simulink model "invBridge120"  (R2026a)
settings: Solver=FixedStepDiscrete  StopTime=0.1  FixedStep=ip.Ts_power
model workspace (MATLAB code in the model file):
  | ip = invParams();
libraries: nesl_utility x18, fl_lib x13, ee_lib x3
settings Model: Creator=phamn  LastModifiedBy=phamn
settings SimscapeCC: SimscapeLogType=none

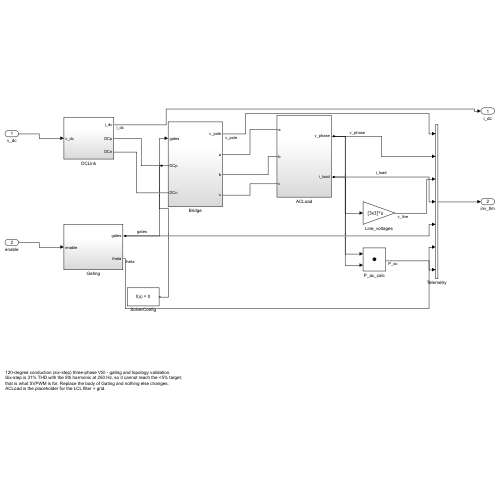
[thumbnail: Simulink's stored preview of the top-level diagram]
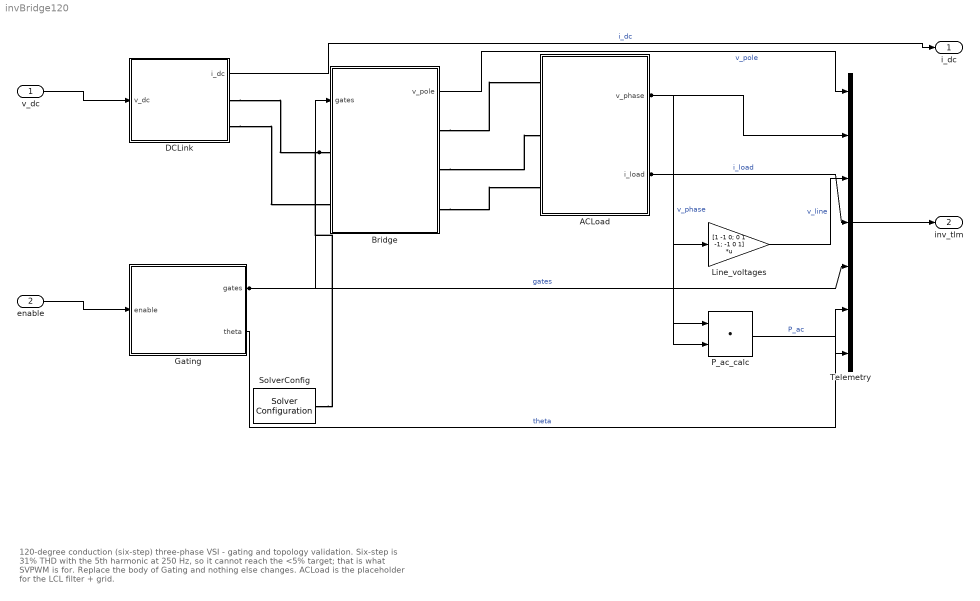
== system invBridge120 ==
  note: 120-degree conduction (six-step) three-phase VSI - gating and topology validation.
      | Six-step is 31% THD with the 5th harmonic at 250 Hz, so it cannot reach the <5% target;
      | that is what SVPWM is for. Replace the body of Gating and nothing else changes.
      | ACLoad is the placeholder for the LCL filter + grid.
  v_dc : Inport
  enable : Inport  Port=2
  ACLoad : Subsystem
  Bridge : Subsystem
  DCLink : Subsystem
  Gating : Subsystem
  Line_voltages : Gain  Gain=[1 -1 0; 0 1 -1; -1 0 1]  Multiplication=Matrix(K*u)
  P_ac_calc : DotProduct  OutDataTypeStr=Inherit: Inherit via internal rule
  SolverConfig : nesl_utility/Solver Configuration  PhysicalDomain=network_engine_domain  SubClassName=solver  LeftPortType=input  RightPortType=generic  Tones=[]  Harmonics=[]  SimulateNoise=off  Profile=off  UseLocalSampling=off  EnableSwitchedLinearOptims=on  FrequencyDomain=off  UseCCode=off  RelTol=0.001  AbsTol=0.001  MinStep=1e-09  ToWorkspace=off  RevertToSquareIcSolve=off  NumHomotopyIterations=100  PhasorMode=off  PhasorModeNumHarmonics=1  ConsistencySolver=NEWTON_XTOL_AFTER_FTOL  CanonicalOrdering=CANONICAL  OptimizeIntermediates=OPTIMIZED  IndexReductionMethod=DerivativeReplacement  DoDC=off  ResidualTolerance=1e-09  ConsistencyTolSource=GLOBAL  ConsistencyAbsTol=0.001  ConsistencyRelTol=0.001  ConsistencyTolFactor=0.001  UseLocalSolver=on  LocalSolverChoice=NE_BACKWARD_EULER_ADVANCER  ResolveIndetEquations=on  FunctionEvalNumThread=1  LocalSolverSampleTime=ip.Ts_power  DoFixedCost=off  MaxNonlinIter=3  MaxModeIter=2  ComputeImpulses=off  ImpulseIterations=2  LinearAlgebra=auto  LinearAlgebraNumThread=0  EquationFormulation=NE_TIME_EF  DelaysMemoryBudget=1024  AutomaticFiltering=on  FilteringTimeConstant=0.001  PartitionStorageMethod=AS_NEEDED  PartitionMemoryBudget=1024  PartitionMethod=ROBUST  MultibodyUseLocalSolver=off  MultibodyLocalSolverChoice=ODE1  MultibodyLocalSolverSampleTime=0.001
  Telemetry : BusCreator  Inputs=7
  i_dc : Outport
  inv_tlm : Outport  Port=2
  wires:
  v_dc/1 -> DCLink/1(v_dc)
  enable/1 -> Gating/1(enable)
  Gating/1(gates) -> Bridge/1(gates), Telemetry/5  "gates"
  Gating/2(theta) -> Telemetry/6  "theta"
  Bridge/1(v_pole) -> Telemetry/1  "v_pole"
  ACLoad/1(v_phase) -> Telemetry/2, Line_voltages/1, P_ac_calc/1  "v_phase"
  ACLoad/2(i_load) -> Telemetry/4, P_ac_calc/2  "i_load"
  Line_voltages/1 -> Telemetry/3  "v_line"
  P_ac_calc/1 -> Telemetry/7  "P_ac"
  DCLink/1(i_dc) -> i_dc/1  "i_dc"
  Telemetry/1 -> inv_tlm/1
  connections:
  Bridge/LConn1 -- DCLink/RConn1 -- SolverConfig/RConn1
  DCLink/RConn2 -- Bridge/LConn2
  Bridge/RConn1 -- ACLoad/LConn1
  Bridge/RConn2 -- ACLoad/LConn2
  Bridge/RConn3 -- ACLoad/LConn3

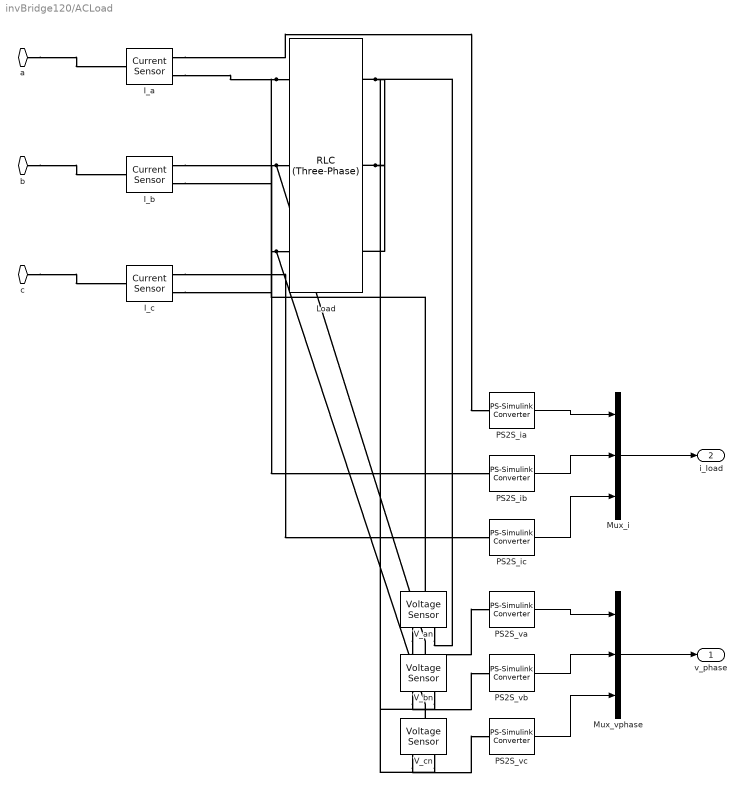
== system invBridge120/ACLoad ==
  I_a : fl_lib/Electrical/Electrical Sensors/Current Sensor
  I_b : fl_lib/Electrical/Electrical Sensors/Current Sensor
  I_c : fl_lib/Electrical/Electrical Sensors/Current Sensor
  Load : ee_lib/Passive/RLC Assemblies/RLC (Three-Phase)  port_option=ee.enum.threePhasePort.expanded  component_structure=ee.enum.rlc.structure.R  R=ip.R_load Ohm  L=ip.L_load H  C=ip.Cf F  R_parasitic=0 Ohm  G_parasitic=0 1/Ohm  IL_specify=off  IL_priority=High  IL=[0, 0, 0] A  IL_nominal_specify=off  IL_nominal_value=1  IL_nominal_unit=A  VC_specify=off  VC_priority=High  VC=[0, 0, 0] V  VC_nominal_specify=off  VC_nominal_value=1  VC_nominal_unit=V
  Mux_i : Mux  Inputs=3
  Mux_vphase : Mux  Inputs=3
  PS2S_ia : nesl_utility/PS-Simulink Converter  PhysicalDomain=network_engine_domain  SubClassName=ps_output  LeftPortType=input  RightPortType=output  PseudoPeriodic=off  Frequencies=[]  VectorFormat=inherit  Unit=inherit  AffineConversion=off
  PS2S_ib : nesl_utility/PS-Simulink Converter  PhysicalDomain=network_engine_domain  SubClassName=ps_output  LeftPortType=input  RightPortType=output  PseudoPeriodic=off  Frequencies=[]  VectorFormat=inherit  Unit=inherit  AffineConversion=off
  PS2S_ic : nesl_utility/PS-Simulink Converter  PhysicalDomain=network_engine_domain  SubClassName=ps_output  LeftPortType=input  RightPortType=output  PseudoPeriodic=off  Frequencies=[]  VectorFormat=inherit  Unit=inherit  AffineConversion=off
  PS2S_va : nesl_utility/PS-Simulink Converter  PhysicalDomain=network_engine_domain  SubClassName=ps_output  LeftPortType=input  RightPortType=output  PseudoPeriodic=off  Frequencies=[]  VectorFormat=inherit  Unit=inherit  AffineConversion=off
  PS2S_vb : nesl_utility/PS-Simulink Converter  PhysicalDomain=network_engine_domain  SubClassName=ps_output  LeftPortType=input  RightPortType=output  PseudoPeriodic=off  Frequencies=[]  VectorFormat=inherit  Unit=inherit  AffineConversion=off
  PS2S_vc : nesl_utility/PS-Simulink Converter  PhysicalDomain=network_engine_domain  SubClassName=ps_output  LeftPortType=input  RightPortType=output  PseudoPeriodic=off  Frequencies=[]  VectorFormat=inherit  Unit=inherit  AffineConversion=off
  V_an : fl_lib/Electrical/Electrical Sensors/Voltage Sensor
  V_bn : fl_lib/Electrical/Electrical Sensors/Voltage Sensor
  V_cn : fl_lib/Electrical/Electrical Sensors/Voltage Sensor
  a : PMIOPort  Side=Left
  b : PMIOPort  Port=2  Side=Left
  c : PMIOPort  Port=3  Side=Left
  v_phase : Outport
  i_load : Outport  Port=2
  wires:
  PS2S_ia/1 -> Mux_i/1
  PS2S_va/1 -> Mux_vphase/1
  PS2S_ib/1 -> Mux_i/2
  PS2S_vb/1 -> Mux_vphase/2
  PS2S_ic/1 -> Mux_i/3
  PS2S_vc/1 -> Mux_vphase/3
  Mux_i/1 -> i_load/1
  Mux_vphase/1 -> v_phase/1
  connections:
  a/RConn1 -- I_a/LConn1
  Load/LConn1 -- I_a/RConn2 -- V_an/LConn1
  I_a/RConn1 -- PS2S_ia/LConn1
  V_an/RConn2 -- V_bn/RConn2 -- V_cn/RConn2 -- Load/RConn1 -- Load/RConn2 -- Load/RConn3
  V_an/RConn1 -- PS2S_va/LConn1
  b/RConn1 -- I_b/LConn1
  Load/LConn2 -- I_b/RConn2 -- V_bn/LConn1
  I_b/RConn1 -- PS2S_ib/LConn1
  V_bn/RConn1 -- PS2S_vb/LConn1
  c/RConn1 -- I_c/LConn1
  Load/LConn3 -- I_c/RConn2 -- V_cn/LConn1
  I_c/RConn1 -- PS2S_ic/LConn1
  V_cn/RConn1 -- PS2S_vc/LConn1

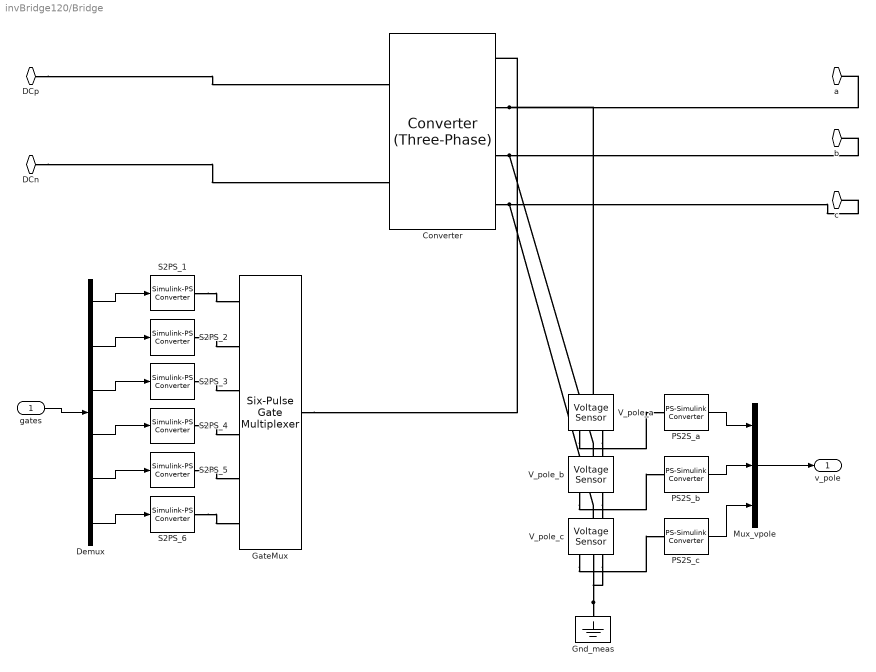
== system invBridge120/Bridge ==
  gates : Inport
  Converter : ee_lib/Semiconductors & Converters/Converters/Converter (Three-Phase)  port_option=ee.enum.threePhasePort.expanded  fidelity_option=ee.enum.converters.fidelity.detailed  device_type=ee.enum.converters.switchingdevice.igbt  showThermalPort=false  K=0  Vth=ip.Vth_gate V  Vgt=1 V  Vgt_off=-1 V  Ih=1 A  Vf=ip.Vf_dev V  Ron=ip.Ron_dev Ohm  Rds=0.001 Ohm  Goff=ip.Goff_dev 1/Ohm  Eon_scalar=22.86e-3 J  Eoff_scalar=17.14e-3 J  Eoff_natural_commutation=10e-3 J  Voff=300 V  Iout_scalar=600 A  onCurrentMeasDelay=0 s  useCurrentFromPreviousCycle=false  useVoltageFromPreviousCycle=false  diode_param=ee.enum.converters.protectiondiode.nodynamics  diode_Vf=ip.Vf_dev V  diode_Ron=ip.Ron_dev Ohm  diode_Goff=1e-5 1/Ohm  diode_C=50 nF  diode_iRM=-235 A  diode_iF=300 A  diode_idot=-50 A/us  diode_trr_param=ee.enum.converters.diodetrr.trr_factor  diode_trr_factor=3  diode_trr=15 us  diode_Qrr=1500 s*uA  diode_rec_loss_model=ee.enum.diode.reverseRecoveryModel.fixed  diode_ErecVal=0 J  diode_scaleWithIandV=false  diode_ErecMat=zeros(2, 3) J  diode_TjrecVec=[298.15, 398.15] K  diode_IfrecVec=[.1, 1, 10] A  diode_IrecVal=10 A  diode_VrecVal=10 V  diode_tFilter=1 / 1000 / 100 s  thermal_network_parameterization=ee.enum.thermalNetworkTopology.external  Rth=[.08, .5] K/W  Rth_Cauer=[.08, .1, .5] K/W  Rth_Foster=[.08, .14, .22, .16] K/W  thermal_mass_parameterization=ee.enum.thermalNetwork.timeconstant  thermal_mass=[.01, .5] J/K  thermal_mass_Cauer=[.01, .1, .5] J/K  thermal_mass_Foster=[.001, .005, .05, .5] J/K  thermal_time_constant=[.001, .2] s  thermal_time_constant_Cauer=[.001, .1, .2] s  thermal_time_constant_Foster=[7e-05, .0007, .01, .08] s  thermal_mass_initial_temperatures=[25, 25] degC  thermal_mass_initial_temperatures_Cauer=[25, 25, 25] degC  junction_thermal_mass=0.01 J/K  Tvec_initial_Foster=[25, 25, 25, 25] degC  snubber_type=ee.enum.converters.snubber.exclude  Cs=1e-7 F  Rs=0.1 Ohm  Vce_loss=[0, 150, 300] V
  Demux : Demux  Outputs=6
  GateMux : ee_lib/Semiconductors & Converters/Converters/Six-Pulse Gate Multiplexer  port_option=ee.enum.controlport.ps
  Gnd_meas : fl_lib/Electrical/Electrical Elements/Electrical Reference
  Mux_vpole : Mux  Inputs=3
  PS2S_a : nesl_utility/PS-Simulink Converter  PhysicalDomain=network_engine_domain  SubClassName=ps_output  LeftPortType=input  RightPortType=output  PseudoPeriodic=off  Frequencies=[]  VectorFormat=inherit  Unit=inherit  AffineConversion=off
  PS2S_b : nesl_utility/PS-Simulink Converter  PhysicalDomain=network_engine_domain  SubClassName=ps_output  LeftPortType=input  RightPortType=output  PseudoPeriodic=off  Frequencies=[]  VectorFormat=inherit  Unit=inherit  AffineConversion=off
  PS2S_c : nesl_utility/PS-Simulink Converter  PhysicalDomain=network_engine_domain  SubClassName=ps_output  LeftPortType=input  RightPortType=output  PseudoPeriodic=off  Frequencies=[]  VectorFormat=inherit  Unit=inherit  AffineConversion=off
  S2PS_{1..6} (6 alike) : nesl_utility/Simulink-PS Converter  PhysicalDomain=network_engine_domain  SubClassName=ps_input  LeftPortType=input  RightPortType=output  PseudoPeriodic=off  Frequencies=[]  NoiseDistribution=none  NoiseParameters=[]  Unit=1  AffineConversion=off  FilteringAndDerivatives=provide  SimscapeFilterOrder=1  InputFilterTimeConstant=0.001  UdotUserProvided=0
  V_pole_a : fl_lib/Electrical/Electrical Sensors/Voltage Sensor
  V_pole_b : fl_lib/Electrical/Electrical Sensors/Voltage Sensor
  V_pole_c : fl_lib/Electrical/Electrical Sensors/Voltage Sensor
  DCp : PMIOPort  Side=Left
  DCn : PMIOPort  Port=2  Side=Left
  a : PMIOPort  Port=3  Side=Right
  b : PMIOPort  Port=4  Side=Right
  c : PMIOPort  Port=5  Side=Right
  v_pole : Outport
  wires:
  Demux/1 -> S2PS_1/1
  Demux/2 -> S2PS_2/1
  Demux/3 -> S2PS_3/1
  Demux/4 -> S2PS_4/1
  Demux/5 -> S2PS_5/1
  Demux/6 -> S2PS_6/1
  gates/1 -> Demux/1
  PS2S_a/1 -> Mux_vpole/1
  PS2S_b/1 -> Mux_vpole/2
  PS2S_c/1 -> Mux_vpole/3
  Mux_vpole/1 -> v_pole/1
  connections:
  S2PS_1/RConn1 -- GateMux/LConn1
  S2PS_2/RConn1 -- GateMux/LConn2
  S2PS_3/RConn1 -- GateMux/LConn3
  S2PS_4/RConn1 -- GateMux/LConn4
  S2PS_5/RConn1 -- GateMux/LConn5
  S2PS_6/RConn1 -- GateMux/LConn6
  GateMux/RConn1 -- Converter/LConn1
  DCp/RConn1 -- Converter/RConn1
  DCn/RConn1 -- Converter/RConn2
  a/RConn1 -- Converter/LConn2 -- V_pole_a/LConn1
  V_pole_a/RConn2 -- V_pole_b/RConn2 -- Gnd_meas/LConn1 -- V_pole_c/RConn2
  V_pole_a/RConn1 -- PS2S_a/LConn1
  b/RConn1 -- Converter/LConn3 -- V_pole_b/LConn1
  V_pole_b/RConn1 -- PS2S_b/LConn1
  c/RConn1 -- Converter/LConn4 -- V_pole_c/LConn1
  V_pole_c/RConn1 -- PS2S_c/LConn1

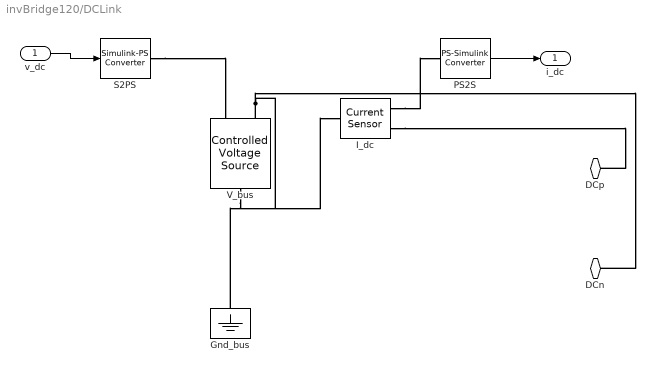
== system invBridge120/DCLink ==
  v_dc : Inport
  Gnd_bus : fl_lib/Electrical/Electrical Elements/Electrical Reference
  I_dc : fl_lib/Electrical/Electrical Sensors/Current Sensor
  PS2S : nesl_utility/PS-Simulink Converter  PhysicalDomain=network_engine_domain  SubClassName=ps_output  LeftPortType=input  RightPortType=output  PseudoPeriodic=off  Frequencies=[]  VectorFormat=inherit  Unit=inherit  AffineConversion=off
  S2PS : nesl_utility/Simulink-PS Converter  PhysicalDomain=network_engine_domain  SubClassName=ps_input  LeftPortType=input  RightPortType=output  PseudoPeriodic=off  Frequencies=[]  NoiseDistribution=none  NoiseParameters=[]  Unit=1  AffineConversion=off  FilteringAndDerivatives=provide  SimscapeFilterOrder=1  InputFilterTimeConstant=0.001  UdotUserProvided=0
  V_bus : fl_lib/Electrical/Electrical Sources/Controlled Voltage Source
  DCp : PMIOPort  Side=Right
  DCn : PMIOPort  Port=2  Side=Right
  i_dc : Outport
  wires:
  v_dc/1 -> S2PS/1
  PS2S/1 -> i_dc/1
  connections:
  S2PS/RConn1 -- V_bus/RConn1
  V_bus/LConn1 -- I_dc/LConn1
  I_dc/RConn2 -- DCp/RConn1
  DCn/RConn1 -- V_bus/RConn2 -- Gnd_bus/LConn1
  I_dc/RConn1 -- PS2S/LConn1

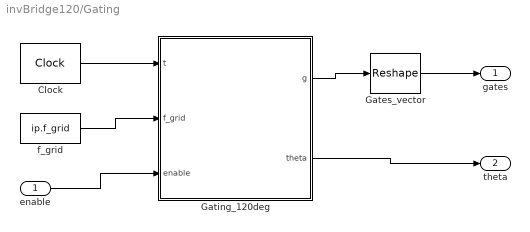
== system invBridge120/Gating ==
  enable : Inport
  Clock : DigitalClock  SampleTime=ip.Ts_power
  Gates_vector : Reshape
  Gating_120deg : MATLAB Function  TreatAsAtomicUnit=on
  f_grid : Constant  Value=ip.f_grid
  gates : Outport
  theta : Outport  Port=2
  wires:
  Clock/1 -> Gating_120deg/1(t)
  f_grid/1 -> Gating_120deg/2(f_grid)
  enable/1 -> Gating_120deg/3(enable)
  Gating_120deg/1(g) -> Gates_vector/1
  Gates_vector/1 -> gates/1
  Gating_120deg/2(theta) -> theta/1

== matlab function invBridge120/Gating/Gating_120deg ==
  data: t input; g output; f_grid input; enable input; theta output
function [g, theta] = gating_120deg(t, f_grid, enable)
%#codegen
% 120-degree conduction gating for a three-phase two-level bridge.
%
% Gate order matches the Six-Pulse Gate Multiplexer: [a+ a- b+ b- c+ c-].
% Verified by firing one gate at a time into a split DC bus, and confirmed
% by the multiplexer port labels Ga(H) Ga(L) Gb(H) Gb(L) Gc(H) Gc(L).
%
% Each device conducts for 120 deg and the two devices of a leg are
% separated by 60 deg of silence, so no dead time is needed here. SPWM
% will need it.
%
% The angles are compared directly rather than built from Pulse Generator
% blocks: 120 deg is 1/3 of the period, which is not an integer number of
% fixed-step samples, and Simulink rejects it. This form is exact at any
% step size, and it is where the carrier comparison goes for SPWM.
theta = mod(360*f_grid*t, 360);                    % electrical angle, deg
g = zeros(6,1);
if enable > 0.5
    g(1) = double(theta >=   0 && theta < 120);    % a+
    g(2) = double(theta >= 180 && theta < 300);    % a-
    g(3) = double(theta >= 120 && theta < 240);    % b+
    g(4) = double(theta >= 300 || theta <  60);    % b-
    g(5) = double(theta >= 240 && theta < 360);    % c+
    g(6) = double(theta >=  60 && theta < 180);    % c-
end
